simulink model "p1_4"  (R2022b)
settings: Solver=VariableStepAuto  StartTime=0.0  StopTime=25.0  RelTol=1e-3
settings Model: Creator=Ausu  LastModifiedBy=Ausu

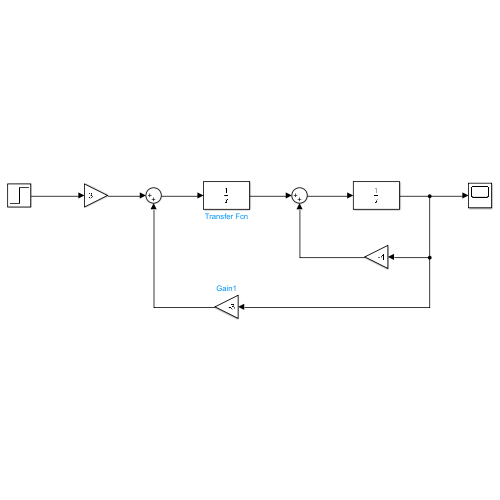
[thumbnail: Simulink's stored preview of the top-level diagram]
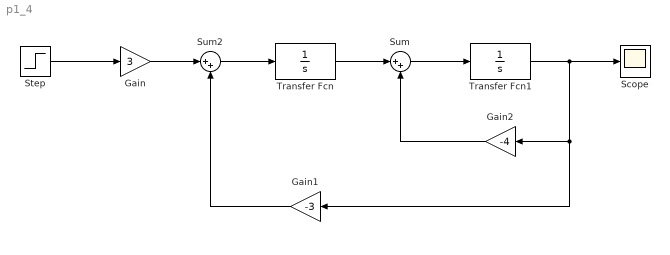
== system p1_4 ==
  Gain : Gain  Gain=3
  Gain1 : Gain  Gain=-3
  Gain2 : Gain  Gain=-4
  Scope : Scope
  Step : Step  Time=0  SampleTime=0
  Sum : Sum  Inputs=|++
  Sum2 : Sum  Inputs=|++
  Transfer Fcn : TransferFcn  Denominator=[1 0]
  Transfer Fcn1 : TransferFcn  Denominator=[1 0]
  wires:
  Step/1 -> Gain/1
  Gain/1 -> Sum2/1
  Sum2/1 -> Transfer Fcn/1
  Gain1/1 -> Sum2/2
  Transfer Fcn/1 -> Sum/1
  Sum/1 -> Transfer Fcn1/1
  Gain2/1 -> Sum/2
  Transfer Fcn1/1 -> Gain1/1, Gain2/1, Scope/1
